simulink model "RD_wLwR"  (R2020b)
settings: Solver=VariableStepAuto  StartTime=0.0  StopTime=100  RelTol=1e-3
values from neighbouring files (symbols this model uses):
  L = 1    [Kinematics_model.m]    (also in Path_Planning.m)
  r_w = 0.2    [Kinematics_model.m]    (also in Path_Planning.m)
  theta0 = 5*pi/180    (= 0.0872664625997)    [Kinematics_model.m]    (also in Path_Planning.m)
  x0 = 0    [Kinematics_model.m]    (also in Path_Planning.m)
  xd = x(length(x))    [APF.m]    (also in Kinematics_model.m = 20; Path_Planning.m = 6)
  y0 = 0    [Kinematics_model.m]    (also in Path_Planning.m)
  yd = y(length(y))    [APF.m]    (also in Kinematics_model.m = 15; Path_Planning.m = 7)
libraries: simulink_extras x1, mobileRoboticsLib x1
settings Model: Creator=Roooooomaaaaaaaaaaaa  LastModifiedBy=Roooooomaaaaaaaaaaaa

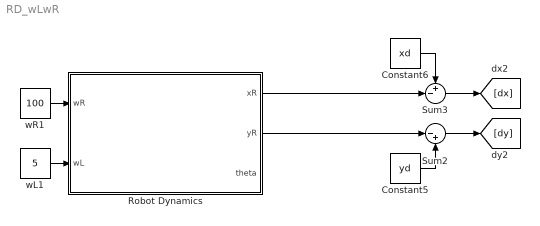
== system RD_wLwR ==
  Constant5 : Constant  Value=yd
  Constant6 : Constant  Value=xd
  Robot Dynamics : Subsystem
  Sum2 : Sum  Inputs=|-+
  Sum3 : Sum  Inputs=+-|
  wL1 : Constant  Value=5
  wR1 : Constant  Value=100
  wires:
  Constant5/1 -> Sum2/2
  wR1/1 -> Robot Dynamics/1(wR)
  Sum3/1 -> [dx]
  Sum2/1 -> [dy]
  Constant6/1 -> Sum3/1
  Robot Dynamics/2(yR) -> Sum2/1
  wL1/1 -> Robot Dynamics/2(wL)
  Robot Dynamics/1(xR) -> Sum3/2

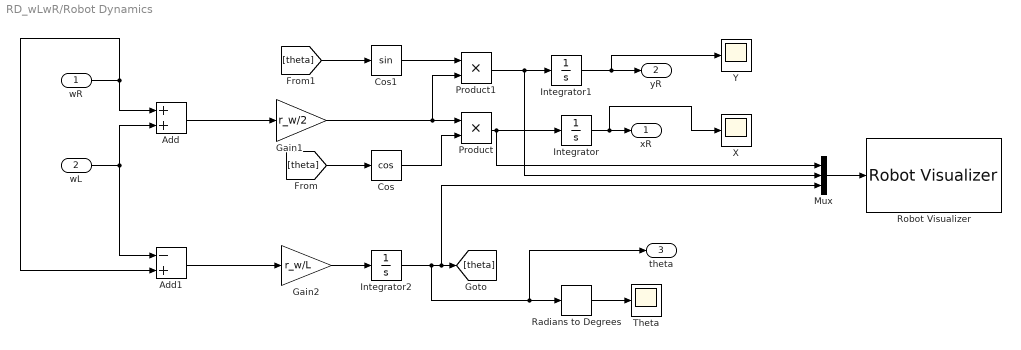
== system RD_wLwR/Robot Dynamics ==
  wR : Inport
  wL : Inport  Port=2
  Add : Sum
  Add1 : Sum  Inputs=-+
  Cos : Trigonometry  Operator=cos
  Cos1 : Trigonometry
  Gain1 : Gain  Gain=r_w/2
  Gain2 : Gain  Gain=r_w/L
  Integrator : Integrator  InitialCondition=x0
  Integrator1 : Integrator  InitialCondition=y0
  Integrator2 : Integrator  InitialCondition=theta0
  Mux : Mux  Inputs=3
  Product : Product
  Product1 : Product
  Radians to Degrees : simulink_extras/Transformations/Radians to Degrees
  Robot Visualizer : mobileRoboticsLib/Environments/Robot Visualizer  robotRadius=r_w  showTrajectory=on  hasWaypoints=off  hasLidar=off  sensorOffset=[ 0, 0 ]  scanAngles=[ -pi/4, 0, pi/4 ]  hasObjDetector=off  objDetectorOffset=[ 0, 0 ]  objDetectorAngle=0  objDetectorFOV=pi/4  objDetectorMaxRange=5  objectColors=[ 1, 0, 0; 0, 1, 0; 0, 0, 1 ]  objectMarkers=s
  Theta : Scope
  X : Scope
  Y : Scope
  xR : Outport
  yR : Outport  Port=2
  theta : Outport  Port=3
  wires:
  Radians to Degrees/1 -> Theta/1
  Integrator1/1 -> Y/1, yR/1
  Cos/1 -> Product/2
  Integrator2/1 -> theta/1, Radians to Degrees/1, Mux/3, [theta]
  Product1/1 -> Mux/2, Integrator1/1
  Cos1/1 -> Product1/1
  Add1/1 -> Gain2/1
  Gain2/1 -> Integrator2/1
  Add/1 -> Gain1/1
  wL/1 -> Add1/1, Add/2
  Integrator/1 -> xR/1, X/1
  Gain1/1 -> Product1/2, Product/1
  wR/1 -> Add1/2, Add/1
  [theta] -> Cos/1
  [theta] -> Cos1/1
  Product/1 -> Mux/1, Integrator/1
  Mux/1 -> Robot Visualizer/1
